simulink model "master_H2_sys"  (R2015a)
settings: Solver=ode45  SolverMode=SingleTasking  StartTime=0.0  StopTime=10.0  RelTol=1e-3
values from neighbouring files (symbols this model uses):
  A = dsys.a    [master_H2.m]    (also in master_H2_decentralized_from_example.m = [a1; a2; a3; a4]; master_disc_H2_feedback.m = A_z; master_disc_H2_feedback_example.m = [a1; a2; a3; a4]; master_h2.m = [0 1; 0 -Bm/Mm])
  Bu = B    [master_H2.m]    (also in master_H2_decentralized_from_example.m = [bu1; bu2; bu3; bu4]; master_disc_H2_feedback.m = B_z; master_disc_H2_feedback_example.m = [bu1; bu2; bu3; bu4])
  K = L_s * inv(X_s)    [master_H2.m]    (also in master_H2_decentralized_from_example.m; master_disc_H2_feedback.m = mat1*mat2*mat3; master_disc_H2_feedback_example.m = mat1*mat2*mat3; master_h2.m = output.P)
settings Model: Creator=enrico-giordano  LastModifiedBy=enrico-giordano
settings OptimizationCC: BlockReduction=off  BooleanDataType=off
settings DebuggingCC: SaveWithParameterizedLinksMsg=none  UnderspecifiedInitializationDetection=Classic  MergeDetectMultiDrivingBlocksExec=none  SignalResolutionControl=TryResolveAllWithWarning
settings HardwareCC: TargetUnknown=on

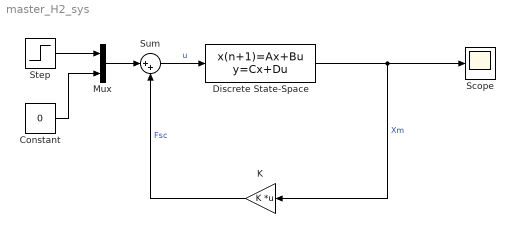
== system master_H2_sys ==
  Constant : Constant  Value=0
  Discrete State-Space : DiscreteStateSpace  A=A  B=Bu  C=eye(size(A,1))  D=zeros(4,2)  SampleTime=0.1
  K : Gain  Gain=K  Multiplication=Matrix(K*u)
  Mux : Mux  Inputs=2
  Scope : Scope
  Step : Step  SampleTime=0
  Sum : Sum  Inputs=|++
  wires:
  Sum/1 -> Discrete State-Space/1  "u"
  K/1 -> Sum/2  "Fsc"
  Discrete State-Space/1 -> K/1, Scope/1  "Xm"
  Mux/1 -> Sum/1
  Step/1 -> Mux/1
  Constant/1 -> Mux/2
